simulink model "Boullis_Eq_Mod"  (R2024b)
settings: Solver=VariableStepAuto  StartTime=0.0  StopTime=10.0  RelTol=1e-3
values from neighbouring files (symbols this model uses):
  p = 1.060    (= 1.06)    [Bernoullis_Equation_Var.m]    (also in Boullis_Equation.m)
  P1 = 16000    [Bernoullis_Equation_Var.m]    (also in Boullis_Equation.m = 725)
  V1 = 0    [Bernoullis_Equation_Var.m]    (also in Boullis_Equation.m)
  V2 = 38    [Bernoullis_Equation_Var.m]    (also in Boullis_Equation.m)
settings Model: Creator=Stephon Woodson  LastModifiedBy=Stephon Woodson

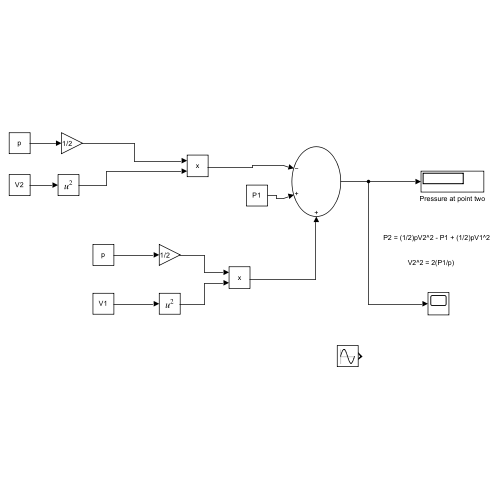
[thumbnail: Simulink's stored preview of the top-level diagram]
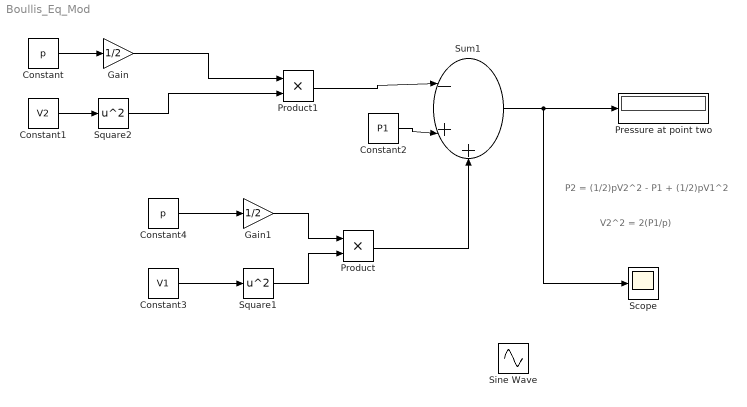
== system Boullis_Eq_Mod ==
  note: P2 = (1/2)pV2^2 - P1 + (1/2)pV1^2
  note: V2^2 = 2(P1/p)
  Constant : Constant  Value=p
  Constant1 : Constant  Value=V2
  Constant2 : Constant  Value=P1
  Constant3 : Constant  Value=V1
  Constant4 : Constant  Value=p
  Gain : Gain  Gain=1/2
  Gain1 : Gain  Gain=1/2
  Pressure at point two : Display
  Product : Product
  Product1 : Product
  Scope : Scope
  Sine Wave : Sin  SampleTime=0
  Square1 : Math  Operator=square
  Square2 : Math  Operator=square
  Sum1 : Sum  Inputs=|-++
  wires:
  Sum1/1 -> Scope/1, Pressure at point two/1
  Constant2/1 -> Sum1/2
  Constant/1 -> Gain/1
  Constant1/1 -> Square2/1
  Constant4/1 -> Gain1/1
  Constant3/1 -> Square1/1
  Gain1/1 -> Product/1
  Square1/1 -> Product/2
  Product/1 -> Sum1/3
  Gain/1 -> Product1/1
  Square2/1 -> Product1/2
  Product1/1 -> Sum1/1
